simulink model "OscillatorAndLockin_DynamicFreqMod"  (R2022b)
settings: Solver=VariableStepAuto  StartTime=0.0  StopTime=0.1  RelTol=1e-3
model workspace: external: MAT-File C:\Users\yoni\Documents\MATLAB\Examples\AFM\Dynamic Mode\sampledistanceLJ.mat (data not in the file)
undefined symbols (not defined in the file or in its folder): D, I, N, P
libraries: simulink x8, slpidlib x3, simulink_extras x1
Description:
  | A model of the workings of "Non-contant AFM (Atomic Force Microscopy)" aka "Dynamic mode AFM" aka "FrequencyModulated AFM" (FM-AFM)
  | 
  | This model contains:
  | a model of an AFM tip made of a tuning fork with tip-sample interaction force  i.e. a damped harmonic oscillator with external forces applied.
  | a model of an "auto-resonance" circuitry. produces positive and negative force pulses at certain phases of the tip's oscillations.
  | a model of a "Lock-in Amplifier" with PLL mechanism that tracks the oscillator frequency.
  | 
  | The oscillator is driven at it's own resonance frequency with a constant amplitude.
  | This is done by a controlled positive feedback loop, Autoresonance's force is amplified by a value designed to keep amplitude constant.
  | (using a PID and the Lock-in amplitude estimation)
  | 
  | The lock-in and PLL model uses the lock-in calculated phase and use that value to correct the lock-in's internal frequency
  | so it will match the external oscillator's frequency. (using another PID)
settings Model: PacingRate=1000  VariantFading=off  Creator=Yoni Cohen  LastModifiedBy=yoni
settings ConfigSet: Description=Current Conf
settings SolverCC: AlgebraicLoopSolver=LineSearch
settings DebuggingCC: UnconnectedInputMsg=warning  UnconnectedOutputMsg=warning  UnconnectedLineMsg=warning  UniqueDataStoreMsg=error  SFMachineParentedDataDiag=warning
settings HardwareCC: TargetBitPerPointer=64  TargetBitPerSizeT=64  TargetBitPerPtrDiffT=64  TargetLargestAtomicFloat=Float  TargetIntDivRoundTo=Zero  TargetEndianess=LittleEndian  TargetWordSize=64  TargetHWDeviceType=Intel->x86-64 (Windows64)  ProdEqTarget=off
settings ModelReferenceCC: EnableRefExpFcnMdlSchedulingChecks=on
settings SFSimCC: CustomCodeUndefinedFunction=UseInterfaceOnly

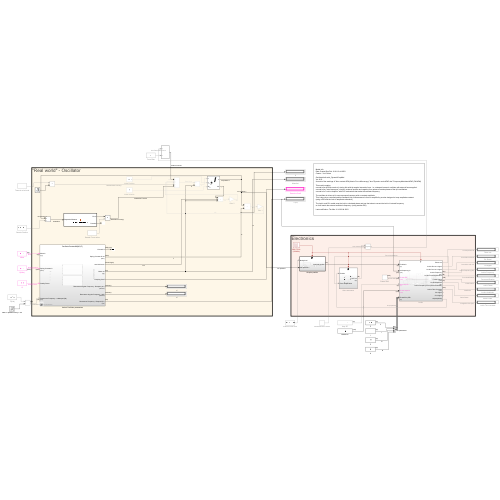
[thumbnail: Simulink's stored preview of the top-level diagram]
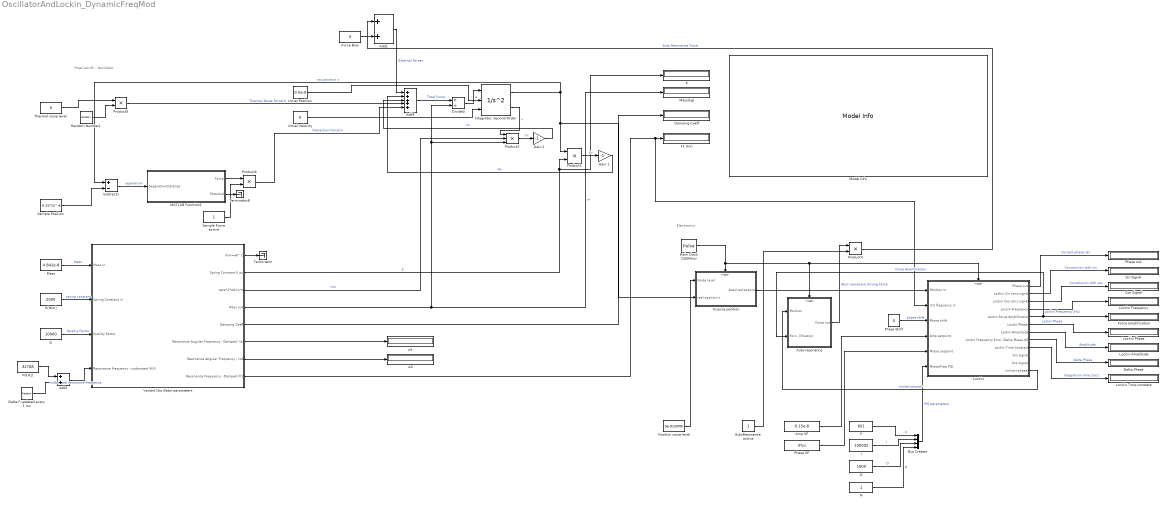
== system OscillatorAndLockin_DynamicFreqMod ==
  note: "Real world" - Oscillator
  note: Electronics
  Acquire position : Subsystem
  Add1 : Sum
  Add2 : Sum
  Add4 : Sum  Inputs=+++++
  Amp SP : Constant  Value=0.15e-8  VectorParams1D=off  SampleTime=-1
  Auto-resonance : Subsystem
  AutoResonance active : Constant  SampleTime=-1
  Bus Creator : BusCreator  Inputs=P,I,D,N
  Cos Signal : Display
  D : Constant  Value=1600  SampleTime=-1
  Damping Coeff : Display
  Delta F updated every 1 ms : RandomNumber  Variance=10  Seed=7546745  SampleTime=1e-3
  Delta Phase : Display
  Divide3 : Product  Inputs=*/
  F0(Hz) : Constant  Value=32768  SampleTime=-1
  F1 (Hz) : Display
  Force Bias : Constant  Value=0  VectorParams1D=off  SampleTime=-1
  Force amplification : Display
  Gain 1 : Gain  Gain=-1
  Gain 2 : Gain  Gain=-1
  I : Constant  Value=100002  SampleTime=-1
  Initial Position : Constant  Value=0.5e-9  VectorParams1D=off
  Initial Velocity : Constant  Value=0
  "Integrator, Second-Order" : SecondOrderIntegrator  ICSourceX=external  LimitX=on  UpperLimitX=0.01  LowerLimitX=-0.01  ICSourceDXDT=external
  K : Display
  K(N/m) : Constant  Value=2000
  Lockin : Subsystem
  Lockin Amplitude : Display
  Lockin Frequency : Display
  Lockin Phase : Display
  Lockin Time constant : Display
  MATLAB Function1 : MATLAB Function  TreatAsAtomicUnit=on
  Main Clock (100MHz) : DiscretePulseGenerator  PulseType=Time based  Period=10^-8  PulseWidth=50
  Mass : Constant  Value=4.842e-8
  Mass(kg) : Display
  Model Info : simulink/Model-Wide Utilities/Model Info  Frame=on  DisplayStringWithTags=|  HorizontalTextAlignment=Left  LeftAlignmentValue=0.02
      | Model Info
      | Date Created %<Created>
      | Creator : %<Creator>
      | %<ModifiedComment>
      | %<ModelName> 
      | Ver. %<ModelVersion>
      | %<Description>
      | Last modification: %<LastModificationDate>
  N : Constant  SampleTime=-1
  P : Constant  Value=601  SampleTime=-1
  Phase SP : Constant  Value=0*pi  SampleTime=-1
  Phase Shift : Constant  Value=0  VectorParams1D=off  SampleTime=-1
  Phase out : Display
  Position noise level : Constant  Value=0e-9/10000  VectorParams1D=off  SampleTime=-1
  Product{1,4..6} (4 alike) : Product
  Product2 : Product  Inputs=3
  Q : Constant  Value=10000
  Random Number1 : RandomNumber  Seed=754666  SampleTime=10^-8
  Sample Force active : Constant  SampleTime=-1
  Sample Position : Constant  Value=-0.25*10^-6  SampleTime=-1
  Sin Signal : Display
  Subtract1 : Sum  Inputs=+-  OutMin=[0]  RndMeth=Nearest
  Terminator : Terminator
  Terminator8 : Terminator
  Thermal noise level : Constant  Value=0  VectorParams1D=off  SampleTime=-1
  Variant Oscillator parameters : Subsystem  Variant=on  VariantControlMode=label  LabelModeActiveChoice=OscillatorTypeVar==1  PropagateVariantConditions=on
  w0 : Display
  w1 : Display
  wires:
  "Integrator, Second-Order"/1 -> Acquire position/2(real position x), Product1/1, Subtract1/1  "osc position x"
  "Integrator, Second-Order"/2 -> Product2/1  "v"
  Product2/1 -> Gain 2/1  "Cv"
  Product1/1 -> Gain 1/1  "Kx"
  Initial Position/1 -> "Integrator, Second-Order"/2
  Initial Velocity/1 -> "Integrator, Second-Order"/3
  Main Clock (100MHz)/1 -> Lockin/Trigger, Auto-resonance/Trigger, Acquire position/Trigger
  Divide3/1 -> "Integrator, Second-Order"/1  "a"
  Auto-resonance/1(Force out) -> Product4/1  "Auto resosnace driving Force"
  Phase Shift/1 -> Lockin/3(Phase shift)  "phase shift"
  Amp SP/1 -> Lockin/4(Amp setpoint)
  F0(Hz)/1 -> Add2/1
  Lockin/5(Lockin Force Amplification) -> Auto-resonance/2(Force Amplification), Force amplification/1  "Force Amplification"
  AutoResonance active/1 -> Product4/2
  Random Number1/1 -> Product5/2
  Thermal noise level/1 -> Product5/1
  Product5/1 -> Add4/4  "Thermal Noise Force(t)"
  Add1/1 -> Add4/1  "External Forces"
  Sample Force active/1 -> Product6/2
  MATLAB Function1/1(Force) -> Product6/1
  Product6/1 -> Add4/5  "Interaction Force(x)"
  Subtract1/1 -> MATLAB Function1/1(SeparationDistance)  "separation"
  K(N/m)/1 -> Variant Oscillator parameters/2(Spring Constant in)  "spring constant"
  Q/1 -> Variant Oscillator parameters/3(Quality Factor)  "Quality Factor"
  Add2/1 -> Variant Oscillator parameters/4(Resonance Frequency - undamped (fr0))  "undamped resonance frequence"
  Variant Oscillator parameters/6(Resonance Angular Frequency - Damped- (w1)) -> w1/1
  Variant Oscillator parameters/8(Resonance Frequency - Damped (fr1)) -> Lockin/2(Init frequency in), F1 (Hz)/1
  Variant Oscillator parameters/4(Mass out) -> Product2/3, Divide3/2, Mass(kg)/1  "m"
  Variant Oscillator parameters/2(Spring Constant K out) -> Product1/2, K/1  "K"
  Variant Oscillator parameters/5(Damping Coeff) -> Damping Coeff/1
  Variant Oscillator parameters/3(zeta*2*w0=c/m) -> Product2/2  "c/m"
  Variant Oscillator parameters/7(Resonance Angular Frequency - (w0)) -> w0/1
  Mass/1 -> Variant Oscillator parameters/1(Mass in)  "Mass"
  Add4/1 -> Divide3/1  "Total Force"
  Gain 1/1 -> Add4/2  "-Kx"
  Gain 2/1 -> Add4/3  "-Cv"
  Variant Oscillator parameters/1(K/m=w0^2) -> Terminator/1
  Lockin/1(Phase out) -> Phase out/1  "Current phase val"
  Lockin/3(Lockin Cos conv signal) -> Cos Signal/1  "Convolution with cos"
  Lockin/4(Lockin Frequency) -> Lockin Frequency/1  "Lockin Frequency [Hz]"
  Lockin/6(Lockin Phase) -> Lockin Phase/1  "Lockin Phase"
  Lockin/8(Lockin Frequency Error (Delta Phase diff)) -> Delta Phase/1  "Delta Phase"
  Lockin/9(Lockin Time Constant) -> Lockin Time constant/1  "Integration time [sec]"
  MATLAB Function1/2(Potential) -> Terminator8/1
  Lockin/7(Lockin Amplitude) -> Lockin Amplitude/1  "Amplitude"
  Lockin/2(Lockin Sin conv signal) -> Sin Signal/1  "Convolution with sin"
  Force Bias/1 -> Add1/2
  Delta F updated every 1 ms/1 -> Add2/2
  Sample Position/1 -> Subtract1/2
  Acquire position/1(Acquired position) -> Lockin/1(Position in)
  Position noise level/1 -> Acquire position/1(Noise level)
  Phase SP/1 -> Lockin/5(Phase setpoint)
  I/1 -> Bus Creator/2  "I"
  D/1 -> Bus Creator/3  "D"
  P/1 -> Bus Creator/1  "P"
  N/1 -> Bus Creator/4  "N"
  Bus Creator/1 -> Lockin/6(Phase/Freq PID)  "PID parameters"
  Lockin/12(sin(wt+phase)) -> Auto-resonance/1(Position)  "sin(wt+phase)"
  Product4/1 -> Add1/1  "Auto Resonance Force"

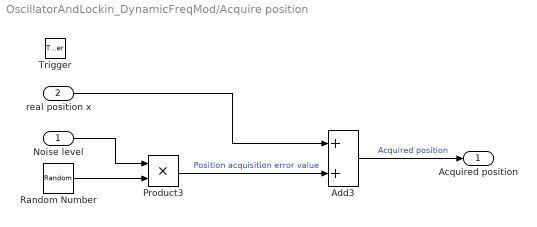
== system OscillatorAndLockin_DynamicFreqMod/Acquire position ==
  Noise level : Inport
  real position x : Inport  Port=2
  Trigger : TriggerPort  VariantControl=Variant  PortDimensions=1
  Add3 : Sum
  Product3 : Product
  Random Number : RandomNumber  Seed=7546767
  Acquired position : Outport  VectorParamsAs1DForOutWhenUnconnected=off
  wires:
  Product3/1 -> Add3/2  "Position acquisition error value"
  Random Number/1 -> Product3/2
  Noise level/1 -> Product3/1
  Add3/1 -> Acquired position/1  "Acquired position"
  real position x/1 -> Add3/1

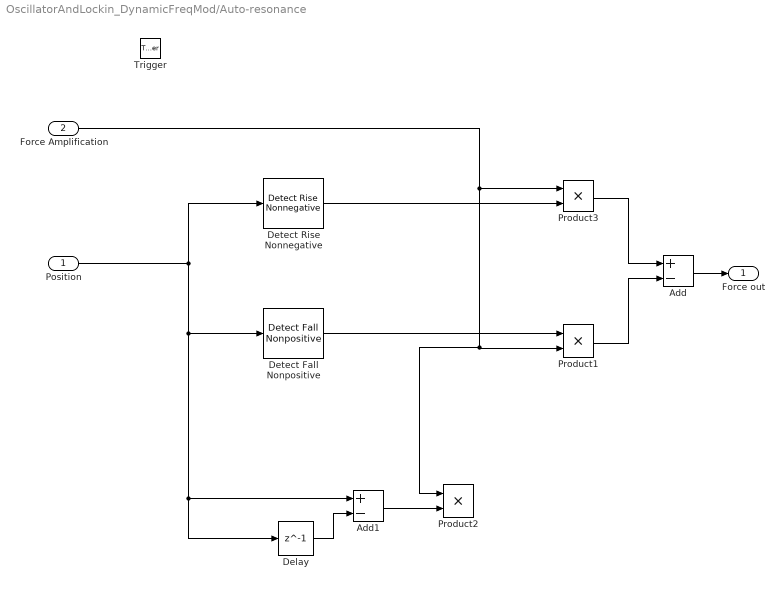
== system OscillatorAndLockin_DynamicFreqMod/Auto-resonance ==
  Position : Inport
  Force Amplification : Inport  Port=2
  Trigger : TriggerPort  VariantControl=Variant  PortDimensions=1
  Add : Sum  Inputs=+-
  Add1 : Sum  Inputs=+-
  Delay : Delay  DelayLength=1  InitialCondition=0
  Detect Fall Nonpositive : simulink/Logic and Bit Operations/Detect Fall Nonpositive  vinit=0  OutDataTypeStr=boolean
  Detect Rise Nonnegative : simulink/Logic and Bit Operations/Detect Rise Nonnegative  vinit=0  OutDataTypeStr=uint8
  Product1 : Product
  Product2 : Product
  Product3 : Product
  Force out : Outport  Unit=N  VectorParamsAs1DForOutWhenUnconnected=off
  wires:
  Position/1 -> Detect Rise Nonnegative/1, Add1/1, Delay/1, Detect Fall Nonpositive/1
  Detect Rise Nonnegative/1 -> Product3/2
  Force Amplification/1 -> Product3/1, Product2/1, Product1/2
  Detect Fall Nonpositive/1 -> Product1/1
  Product1/1 -> Add/2
  Product3/1 -> Add/1
  Delay/1 -> Add1/2
  Add1/1 -> Product2/2
  Add/1 -> Force out/1

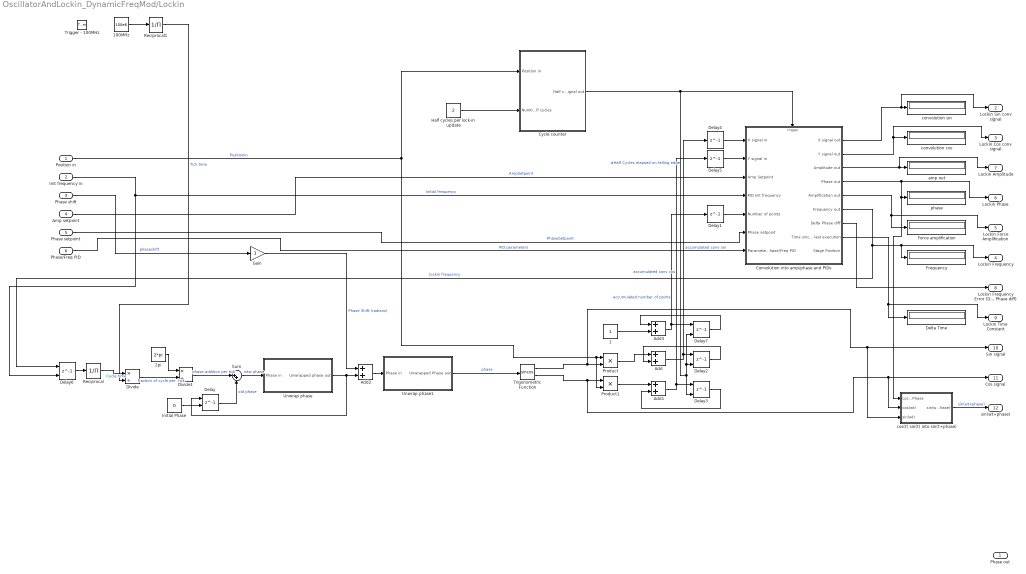
== system OscillatorAndLockin_DynamicFreqMod/Lockin ==
  Position in : Inport  Unit=m
  Init frequency in : Inport  Port=2  Unit=Hz
  Phase shift : Inport  Port=3  OutMin=[-2]  OutMax=[2]  Unit=rad
  Amp setpoint : Inport  Port=4  Unit=m
  Phase setpoint : Inport  Port=5  OutMin=[-2]  OutMax=[2]  Unit=rad
  Phase/Freq PID : Inport  Port=6  Unit=m
  Trigger - 100MHz : TriggerPort  VariantControl=Variant  ShowOutputPort=on  PortDimensions=1
  1 : Constant  OutDataTypeStr=Inherit: Inherit via back propagation
  100MHz : Constant  Value=100e6  OutDataTypeStr=Inherit: Inherit via back propagation
  2pi : Constant  Value=2*pi  OutDataTypeStr=Inherit: Inherit via back propagation
  Add{,1..3} (4 alike) : Sum
  Convolution into amp/phase and PIDs : Subsystem
  Cycle counter : Subsystem
  Delay : Delay  DelayLength=1  InitialConditionSource=Input port  InitialCondition=0
      settings: InputPortMap=u0,p4
  Delay1 : Delay  DelayLength=1  InitialCondition=0
  Delay2 : Delay  DelayLength=1  InitialCondition=0  ExternalReset=Falling
      settings: InputPortMap=u0,r5
  Delay3 : Delay  DelayLength=1  InitialCondition=0  ExternalReset=Falling
      settings: InputPortMap=u0,r5
  Delay4 : Delay  DelayLength=1  InitialCondition=0
  Delay5 : Delay  DelayLength=1  InitialCondition=0
  Delay6 : Delay  DelayLength=1  InitialConditionSource=Input port  InitialCondition=0
      settings: InputPortMap=u0,p4
  Delay7 : Delay  DelayLength=1  InitialCondition=0  ExternalReset=Falling
      settings: InputPortMap=u0,r5
  Delta Time : Display
  Divide : Product  Inputs=*/
  Divide1 : Product  Inputs=*/
  Force amplification : Display
  Frequency : Display
  Gain : Gain
  Half cycles per lock-in update : Constant  Value=2  OutDataTypeStr=Inherit: Inherit via back propagation  SampleTime=-1
  Initial Phase : Constant  Value=0  OutDataTypeStr=Inherit: Inherit via back propagation
  Product : Product
  Product1 : Product
  Reciprocal : Product  Inputs=/
  Reciprocal1 : Product  Inputs=/
  Sum : Sum  Inputs=|++
  Trigonometric Function : Trigonometry  Operator=sincos  ApproximationMethod=CORDIC  NumberOfIterations=64
  Unwrap phase : Subsystem
  Unwrap phase1 : Subsystem
  amp out : Display
  convolution cos : Display
  convolution sin : Display
  cos(t) sin(t) into sin(t+phase) : Subsystem
  phase : Display
  Phase out : Outport  VectorParamsAs1DForOutWhenUnconnected=off
  Lockin Sin conv signal : Outport  Port=2  VectorParamsAs1DForOutWhenUnconnected=off
  Lockin Cos conv signal : Outport  Port=3  VectorParamsAs1DForOutWhenUnconnected=off
  Lockin Frequency : Outport  Port=4  Unit=Hz  InitialOutput=[32769]  VectorParamsAs1DForOutWhenUnconnected=off
  Lockin Force Amplification : Outport  Port=5  VectorParamsAs1DForOutWhenUnconnected=off
  Lockin Phase : Outport  Port=6  Unit=rad  VectorParamsAs1DForOutWhenUnconnected=off
  Lockin Amplitude : Outport  Port=7  Unit=m  VectorParamsAs1DForOutWhenUnconnected=off
  Lockin Frequency Error (Delta Phase diff) : Outport  Port=8  VectorParamsAs1DForOutWhenUnconnected=off
  Lockin Time Constant : Outport  Port=9  Unit=sec  VectorParamsAs1DForOutWhenUnconnected=off
  Sin signal : Outport  Port=10  VectorParamsAs1DForOutWhenUnconnected=off
  Cos signal : Outport  Port=11  VectorParamsAs1DForOutWhenUnconnected=off
  sin(wt+phase) : Outport  Port=12  VectorParamsAs1DForOutWhenUnconnected=off
  wires:
  Divide/1 -> Divide1/2  "fraction of cycle per  tick"
  2pi/1 -> Divide1/1
  Reciprocal/1 -> Divide/1  "Cycle time"
  Trigonometric Function/1 -> Product/2, cos(t) sin(t) into sin(t+phase)/3(sin(wt)), Sin signal/1
  Trigonometric Function/2 -> Product1/1, cos(t) sin(t) into sin(t+phase)/2(cos(wt)), Cos signal/1
  Reciprocal1/1 -> Divide/2  "Tick time"
  Position in/1 -> Cycle counter/1(Position in), Product1/2, Product/1  "Positionin"
  Delay3/1 -> Add1/2
  Delay/1 -> Sum/2  "old phase"
  Delay2/1 -> Add/2
  Convolution into amp/phase and PIDs/3(Amplitude out) -> Lockin Amplitude/1, amp out/1
  Convolution into amp/phase and PIDs/1(X signal out) -> convolution sin/1, Lockin Sin conv signal/1
  Convolution into amp/phase and PIDs/2(Y signal out) -> Lockin Cos conv signal/1, convolution cos/1
  Add/1 -> Delay4/1, Delay2/1  "accumulated conv sin"
  Add1/1 -> Delay3/1, Delay5/1  "accumulated conv cos"
  Divide1/1 -> Sum/1  "phase addition per tick"
  Amp setpoint/1 -> Convolution into amp/phase and PIDs/3(Amp Setpoint)  "AmpSetpoint"
  Convolution into amp/phase and PIDs/5(Amplification out) -> Lockin Force Amplification/1, Force amplification/1
  Init frequency in/1 -> Delay6/2, Convolution into amp/phase and PIDs/4(PID Init frequency)  "Initial frequency"
  Delay6/1 -> Reciprocal/1
  Unwrap phase/1(Unwrapped phase out) -> Delay/1, Add2/2
  Sum/1 -> Unwrap phase/1(Phase in)  "new phase"
  Add2/1 -> Unwrap phase1/1(Phase in)
  Unwrap phase1/1(Unwrapped Phase out) -> Trigonometric Function/1  "phase"
  Half cycles per lock-in update/1 -> Cycle counter/2(Number of half cycles)
  Gain/1 -> Add2/1  "Phase Shift (radians)"
  Convolution into amp/phase and PIDs/4(Phase out) -> Lockin Phase/1, cos(t) sin(t) into sin(t+phase)/1(Lockin Phase), phase/1
  Convolution into amp/phase and PIDs/6(Frequency out) -> Delay6/1, Frequency/1, Lockin Frequency/1  "lockin frequency"
  Convolution into amp/phase and PIDs/7(Delta Phase diff) -> Lockin Frequency Error (Delta Phase diff)/1
  Convolution into amp/phase and PIDs/8(Time since last execution) -> Lockin Time Constant/1, Delta Time/1
  Product1/1 -> Add1/1
  Product/1 -> Add/1
  Delay5/1 -> Convolution into amp/phase and PIDs/2(Y signal in)
  Delay4/1 -> Convolution into amp/phase and PIDs/1(X signal in)
  Cycle counter/1(Half cycle counter signal out) -> Convolution into amp/phase and PIDs/Trigger, Delay7/2, Delay2/2, Delay3/2  "#Half Cycles elapsed on falling edge"
  Add3/1 -> Delay1/1, Delay7/1  "accumulated number of points"
  Delay7/1 -> Add3/1
  1/1 -> Add3/2
  Delay1/1 -> Convolution into amp/phase and PIDs/5(Number of points)
  Phase shift/1 -> Gain/1  "phaseshift"
  Phase setpoint/1 -> Convolution into amp/phase and PIDs/6(Phase setpoint)  "PhaseSetpoint"
  100MHz/1 -> Reciprocal1/1
  Phase/Freq PID/1 -> Convolution into amp/phase and PIDs/7(Parameters Phase/Freq PID)  "PID parameters"
  Initial Phase/1 -> Delay/2
  cos(t) sin(t) into sin(t+phase)/1(sin(wt+phase)) -> sin(wt+phase)/1  "sin(wt+phase)"

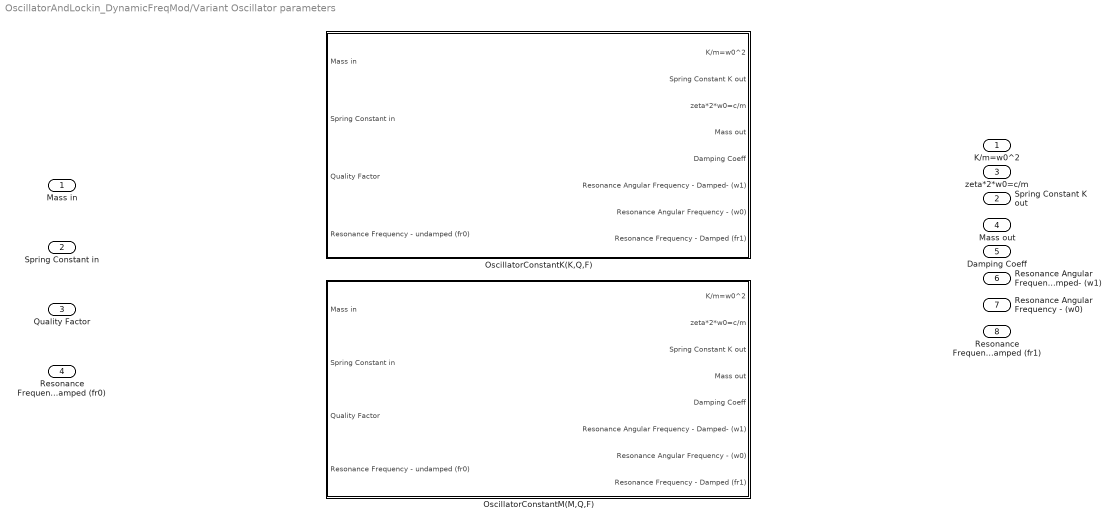
== system OscillatorAndLockin_DynamicFreqMod/Variant Oscillator parameters ==
  Mass in : Inport  Unit=kg
  Spring Constant in : Inport  Port=2  Unit=N/m
  Quality Factor : Inport  Port=3
  Resonance Frequency - undamped (fr0) : Inport  Port=4  Unit=Hz
  OscillatorConstantK(K,Q,F) : Subsystem  VariantControl=OscillatorTypeVar==0
  OscillatorConstantM(M,Q,F) : Subsystem  VariantControl=OscillatorTypeVar==1
  K/m=w0^2 : Outport  VectorParamsAs1DForOutWhenUnconnected=off
  Spring Constant K out : Outport  Port=2  Unit=N/m  VectorParamsAs1DForOutWhenUnconnected=off
  zeta*2*w0=c/m : Outport  Port=3  VectorParamsAs1DForOutWhenUnconnected=off
  Mass out : Outport  Port=4  Unit=kg  VectorParamsAs1DForOutWhenUnconnected=off
  Damping Coeff : Outport  Port=5  VectorParamsAs1DForOutWhenUnconnected=off
  Resonance Angular Frequency - Damped- (w1) : Outport  Port=6  Unit=rad/sec  VectorParamsAs1DForOutWhenUnconnected=off
  Resonance Angular Frequency - (w0) : Outport  Port=7  Unit=rad/sec  VectorParamsAs1DForOutWhenUnconnected=off
  Resonance Frequency - Damped (fr1) : Outport  Port=8  Unit=Hz  VectorParamsAs1DForOutWhenUnconnected=off

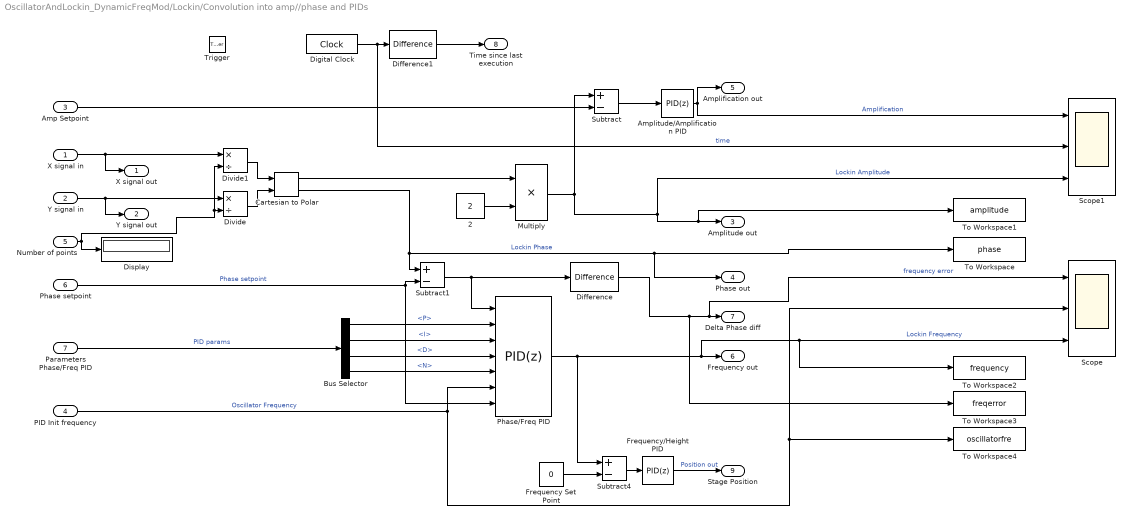
== system OscillatorAndLockin_DynamicFreqMod/Lockin/Convolution into amp//phase and PIDs ==
  X signal in : Inport
  Y signal in : Inport  Port=2
  Amp Setpoint : Inport  Port=3
  PID Init frequency : Inport  Port=4
  Number of points : Inport  Port=5
  Phase setpoint : Inport  Port=6
  Parameters Phase/Freq PID : Inport  Port=7
  Trigger : TriggerPort  TriggerType=falling  VariantControl=Variant  PortDimensions=1
  2 : Constant  Value=2  VectorParams1D=off  SampleTime=-1
  Amplitude/Amplification PID : slpidlib/PID Controller  Controller=PID  Form=Parallel  TimeDomain=Discrete-time  UseExternalTs=off  SampleTime=-1  IntegratorMethod=Trapezoidal  FilterMethod=Trapezoidal  ControllerParametersSource=internal  P=-45000  I=-350000000  UseKiTs=off  D=-10000  N=10  UseFilter=on  TunerSelectOption=Frequency Response Based  InitialConditionSource=internal  InitialConditionForIntegrator=0  InitialConditionForFilter=0  DifferentiatorICPrevScaledInput=0  ExternalReset=none  TrackingMode=off  Kt=1  LimitOutput=off  SatLimitsSource=internal  UpperSaturationLimit=inf  LowerSaturationLimit=-inf  LinearizeAsGain=off  AntiWindupMode=none  Kb=1  LimitIntegrator=off  UpperIntegratorSaturationLimit=inf  LowerIntegratorSaturationLimit=-inf  RndMeth=Round  POutMin=[]  POutMax=[]  IOutMin=[]  IOutMax=[]  DOutMin=[]  DOutMax=[]  NOutMin=[]  NOutMax=[]  SumOutMin=[]  SumOutMax=[]  SaturationOutMin=[]  SaturationOutMax=[]  PParamMin=[]  PParamMax=[]  IParamMin=[]  IParamMax=[]  DParamMin=[]  DParamMax=[]  NParamMin=[]  NParamMax=[]  KbParamMin=[]  KbParamMax=[]  KtParamMin=[]  KtParamMax=[]  KbOutMin=[]  KbOutMax=[]  KtOutMin=[]  KtOutMax=[]  IntegratorOutMin=[]  IntegratorOutMax=[]  FilterOutMin=[]  FilterOutMax=[]  SumI1OutMin=[]  SumI1OutMax=[]  SumI2OutMin=[]  SumI2OutMax=[]  SumI3OutMin=[]  SumI3OutMax=[]  SumI4OutMin=[]  SumI4OutMax=[]  SumDOutMin=[]  SumDOutMax=[]  DifferentiatorOutMin=[]  DifferentiatorOutMax=[]  FilterDiffOutCoefMin=[]  FilterDiffOutCoefMax=[]  ReciprocalOutMin=[]  ReciprocalOutMax=[]  SumDenOutMin=[]  SumDenOutMax=[]  SumNumOutMin=[]  SumNumOutMax=[]  DivideOutMin=[]  DivideOutMax=[]  UdiffTsProdOutMin=[]  UdiffTsProdOutMax=[]  NTsProdOutMin=[]  NTsProdOutMax=[]  UintegralTsProdOutMin=[]  UintegralTsProdOutMax=[]  UngainTsProdOutMin=[]  UngainTsProdOutMax=[]  ClampingZeroOutDataTypeStr=Inherit: Inherit via back propagation  ClampingZeroOutMin=[]  ClampingZeroOutMax=[]  FilterDenConstantOutDataTypeStr=Inherit: Inherit via back propagation  FilterDenConstantOutMin=[]  FilterDenConstantOutMax=[]  PCopyOutDataTypeStr=Inherit: Inherit via back propagation  PCopyOutMin=[]  PCopyOutMax=[]  NCopyOutDataTypeStr=Inherit: Inherit via back propagation  NCopyOutMin=[]  NCopyOutMax=[]  IntegratorContinuousStateAttributes=''  IntegratorStateMustResolveToSignalObject=off  IntegratorRTWStateStorageClass=Auto  FilterContinuousStateAttributes=''  FilterStateMustResolveToSignalObject=off  FilterRTWStateStorageClass=Auto  ParallelPVariant=InternalParameters  IdealPVariant=Disabled  IVariant=InternalParameters  DVariant=InternalParameters  IntegratorVariant=Discrete  SatVariant=Disabled  AWVariant=Passthrough  PCopyVariant=Disabled  TRVariant=Disabled  FdbkBlocksVariant=Forward  IdealPFdbkVariant=Disabled  SatFdbkVariant=Disabled  DerivativeFilterVariant=TrapezoidalFilter  NVariant=InternalParameters  NCopyVariant=InternalParameters  FilterICVariant=InternalICsFilter  IntegratorICVariant=InternalICs  ExternalResetVariant=Disabled  TRSumVariant=Passthrough  SumFdbkVariant=Disabled  SumVariant=Sum_PID  TsampFilterVariant=InternalTs  TsampNgainVariant=Passthrough  TsampIntegralVariant=Passthrough  ExternalSaturationOutDataTypeStr=Inherit: Same as second input
  Bus Selector : BusSelector  OutputSignals=P,I,D,N
  Cartesian to Polar : simulink_extras/Transformations/Cartesian to Polar
  Difference : simulink/Quick Insert/Discrete/Difference  ICPrevInput=0.0  OutMin=[]  OutMax=[]  OutDataType=fixdt(1, 16)  OutScaling=2^-10  DoSatur=off
  Difference1 : simulink/Quick Insert/Discrete/Difference  ICPrevInput=0.0  OutMin=[]  OutMax=[]  OutDataType=fixdt(1, 16)  OutScaling=2^-10  DoSatur=off
  Digital Clock : DigitalClock  SampleTime=-1
  Display : Display
  Divide : Product  Inputs=*/
  Divide1 : Product  Inputs=*/
  Frequency Set Point : Constant  Value=0  SampleTime=-1
  Frequency/Height PID : slpidlib/PID Controller  Controller=PID  Form=Parallel  TimeDomain=Discrete-time  UseExternalTs=off  SampleTime=-1  IntegratorMethod=Forward Euler  FilterMethod=Forward Euler  ControllerParametersSource=internal  P=1  I=1  UseKiTs=off  D=0  N=100  UseFilter=on  TunerSelectOption=Transfer Function Based (PID Tuner App)  InitialConditionSource=internal  InitialConditionForIntegrator=0  InitialConditionForFilter=0  DifferentiatorICPrevScaledInput=0  ExternalReset=none  TrackingMode=off  Kt=1  LimitOutput=off  SatLimitsSource=internal  UpperSaturationLimit=inf  LowerSaturationLimit=-inf  LinearizeAsGain=off  AntiWindupMode=none  Kb=1  LimitIntegrator=off  UpperIntegratorSaturationLimit=inf  LowerIntegratorSaturationLimit=-inf  POutMin=[]  POutMax=[]  IOutMin=[]  IOutMax=[]  DOutMin=[]  DOutMax=[]  NOutMin=[]  NOutMax=[]  SumOutMin=[]  SumOutMax=[]  SaturationOutMin=[]  SaturationOutMax=[]  PParamMin=[]  PParamMax=[]  IParamMin=[]  IParamMax=[]  DParamMin=[]  DParamMax=[]  NParamMin=[]  NParamMax=[]  KbParamMin=[]  KbParamMax=[]  KtParamMin=[]  KtParamMax=[]  KbOutMin=[]  KbOutMax=[]  KtOutMin=[]  KtOutMax=[]  IntegratorOutMin=[]  IntegratorOutMax=[]  FilterOutMin=[]  FilterOutMax=[]  SumI1OutMin=[]  SumI1OutMax=[]  SumI2OutMin=[]  SumI2OutMax=[]  SumI3OutMin=[]  SumI3OutMax=[]  SumI4OutMin=[]  SumI4OutMax=[]  SumDOutMin=[]  SumDOutMax=[]  DifferentiatorOutMin=[]  DifferentiatorOutMax=[]  FilterDiffOutCoefMin=[]  FilterDiffOutCoefMax=[]  ReciprocalOutMin=[]  ReciprocalOutMax=[]  SumDenOutMin=[]  SumDenOutMax=[]  SumNumOutMin=[]  SumNumOutMax=[]  DivideOutMin=[]  DivideOutMax=[]  UdiffTsProdOutMin=[]  UdiffTsProdOutMax=[]  NTsProdOutMin=[]  NTsProdOutMax=[]  UintegralTsProdOutMin=[]  UintegralTsProdOutMax=[]  UngainTsProdOutMin=[]  UngainTsProdOutMax=[]  ClampingZeroOutDataTypeStr=Inherit: Inherit via back propagation  ClampingZeroOutMin=[]  ClampingZeroOutMax=[]  FilterDenConstantOutDataTypeStr=Inherit: Inherit via back propagation  FilterDenConstantOutMin=[]  FilterDenConstantOutMax=[]  PCopyOutDataTypeStr=Inherit: Inherit via back propagation  PCopyOutMin=[]  PCopyOutMax=[]  NCopyOutDataTypeStr=Inherit: Inherit via back propagation  NCopyOutMin=[]  NCopyOutMax=[]  IntegratorContinuousStateAttributes=''  IntegratorStateMustResolveToSignalObject=off  IntegratorRTWStateStorageClass=Auto  FilterContinuousStateAttributes=''  FilterStateMustResolveToSignalObject=off  FilterRTWStateStorageClass=Auto  ParallelPVariant=InternalParameters  IdealPVariant=Disabled  IVariant=InternalParameters  DVariant=InternalParameters  IntegratorVariant=Discrete  SatVariant=Disabled  AWVariant=Passthrough  PCopyVariant=Disabled  TRVariant=Disabled  FdbkBlocksVariant=Forward  IdealPFdbkVariant=Disabled  SatFdbkVariant=Disabled  DerivativeFilterVariant=ForwardEulerFilter  NVariant=InternalParameters  NCopyVariant=Disabled  FilterICVariant=InternalICsFilter  IntegratorICVariant=InternalICs  ExternalResetVariant=Disabled  TRSumVariant=Passthrough  SumFdbkVariant=Disabled  SumVariant=Sum_PID  TsampFilterVariant=InternalTs  TsampNgainVariant=Passthrough  TsampIntegralVariant=Passthrough  ExternalSaturationOutDataTypeStr=Inherit: Same as second input
  Multiply : Product  Inputs=**
  Phase/Freq PID : slpidlib/PID Controller  Controller=PID  Form=Parallel  TimeDomain=Discrete-time  UseExternalTs=off  SampleTime=-1  IntegratorMethod=Forward Euler  FilterMethod=Forward Euler  ControllerParametersSource=external  P=20  I=100  UseKiTs=off  D=1400  N=1  UseFilter=on  TunerSelectOption=Transfer Function Based (PID Tuner App)  InitialConditionSource=external  InitialConditionForIntegrator=0  InitialConditionForFilter=0  DifferentiatorICPrevScaledInput=0  ExternalReset=none  TrackingMode=off  Kt=1  LimitOutput=off  SatLimitsSource=internal  UpperSaturationLimit=inf  LowerSaturationLimit=-inf  LinearizeAsGain=off  AntiWindupMode=none  Kb=1  LimitIntegrator=off  UpperIntegratorSaturationLimit=inf  LowerIntegratorSaturationLimit=-inf  POutMin=[]  POutMax=[]  IOutMin=[]  IOutMax=[]  DOutMin=[]  DOutMax=[]  NOutMin=[]  NOutMax=[]  SumOutMin=[]  SumOutMax=[]  SaturationOutMin=[]  SaturationOutMax=[]  PParamMin=[]  PParamMax=[]  IParamMin=[]  IParamMax=[]  DParamMin=[]  DParamMax=[]  NParamMin=[]  NParamMax=[]  KbParamMin=[]  KbParamMax=[]  KtParamMin=[]  KtParamMax=[]  KbOutMin=[]  KbOutMax=[]  KtOutMin=[]  KtOutMax=[]  IntegratorOutMin=[]  IntegratorOutMax=[]  FilterOutMin=[]  FilterOutMax=[]  SumI1OutMin=[]  SumI1OutMax=[]  SumI2OutMin=[]  SumI2OutMax=[]  SumI3OutMin=[]  SumI3OutMax=[]  SumI4OutMin=[]  SumI4OutMax=[]  SumDOutMin=[]  SumDOutMax=[]  DifferentiatorOutMin=[]  DifferentiatorOutMax=[]  FilterDiffOutCoefMin=[]  FilterDiffOutCoefMax=[]  ReciprocalOutMin=[]  ReciprocalOutMax=[]  SumDenOutMin=[]  SumDenOutMax=[]  SumNumOutMin=[]  SumNumOutMax=[]  DivideOutMin=[]  DivideOutMax=[]  UdiffTsProdOutMin=[]  UdiffTsProdOutMax=[]  NTsProdOutMin=[]  NTsProdOutMax=[]  UintegralTsProdOutMin=[]  UintegralTsProdOutMax=[]  UngainTsProdOutMin=[]  UngainTsProdOutMax=[]  ClampingZeroOutDataTypeStr=Inherit: Inherit via back propagation  ClampingZeroOutMin=[]  ClampingZeroOutMax=[]  FilterDenConstantOutDataTypeStr=Inherit: Inherit via back propagation  FilterDenConstantOutMin=[]  FilterDenConstantOutMax=[]  PCopyOutDataTypeStr=Inherit: Inherit via back propagation  PCopyOutMin=[]  PCopyOutMax=[]  NCopyOutDataTypeStr=Inherit: Inherit via back propagation  NCopyOutMin=[]  NCopyOutMax=[]  IntegratorContinuousStateAttributes=''  IntegratorStateMustResolveToSignalObject=off  IntegratorRTWStateStorageClass=Auto  FilterContinuousStateAttributes=''  FilterStateMustResolveToSignalObject=off  FilterRTWStateStorageClass=Auto  ParallelPVariant=ExternalParameters  IdealPVariant=Disabled  IVariant=ExternalParameters  DVariant=ExternalParameters  IntegratorVariant=Discrete  SatVariant=Disabled  AWVariant=Passthrough  PCopyVariant=Disabled  TRVariant=Disabled  FdbkBlocksVariant=Forward  IdealPFdbkVariant=Disabled  SatFdbkVariant=Disabled  DerivativeFilterVariant=ForwardEulerFilter  NVariant=ExternalParameters  NCopyVariant=Disabled  FilterICVariant=ExternalICs  IntegratorICVariant=ExternalICs  ExternalResetVariant=Disabled  TRSumVariant=Passthrough  SumFdbkVariant=Disabled  SumVariant=Sum_PID  TsampFilterVariant=InternalTs  TsampNgainVariant=Passthrough  TsampIntegralVariant=Passthrough  ExternalSaturationOutDataTypeStr=Inherit: Same as second input
  Scope : Scope  NumInputPorts=3
  Scope1 : Scope  NumInputPorts=3
  Subtract : Sum  Inputs=+-
  Subtract1 : Sum  Inputs=+-
  Subtract4 : Sum  Inputs=+-
  To Workspace : ToWorkspace  VariableName=phase  SaveFormat=Timeseries  SampleTime=-1
  To Workspace1 : ToWorkspace  VariableName=amplitude  SaveFormat=Timeseries  SampleTime=-1
  To Workspace2 : ToWorkspace  VariableName=frequency  SaveFormat=Timeseries  SampleTime=-1
  To Workspace3 : ToWorkspace  VariableName=freqerror  SaveFormat=Timeseries  SampleTime=-1
  To Workspace4 : ToWorkspace  VariableName=oscillatorfre  SaveFormat=Timeseries  SampleTime=-1
  X signal out : Outport  VectorParamsAs1DForOutWhenUnconnected=off
  Y signal out : Outport  Port=2  VectorParamsAs1DForOutWhenUnconnected=off
  Amplitude out : Outport  Port=3  Unit=m  VectorParamsAs1DForOutWhenUnconnected=off
  Phase out : Outport  Port=4  Unit=rad  VectorParamsAs1DForOutWhenUnconnected=off
  Amplification out : Outport  Port=5  Unit=N  VectorParamsAs1DForOutWhenUnconnected=off
  Frequency out : Outport  Port=6  Unit=Hz  InitialOutput=[32766]  VectorParamsAs1DForOutWhenUnconnected=off
  Delta Phase diff : Outport  Port=7  Unit=rad  VectorParamsAs1DForOutWhenUnconnected=off
  Time since last execution : Outport  Port=8  Unit=sec  VectorParamsAs1DForOutWhenUnconnected=off
  Stage Position : Outport  Port=9  Unit=m  VectorParamsAs1DForOutWhenUnconnected=off
  wires:
  X signal in/1 -> Divide1/1, X signal out/1
  Y signal in/1 -> Divide/1, Y signal out/1
  Amp Setpoint/1 -> Subtract/2
  Phase/Freq PID/1 -> Frequency out/1, To Workspace2/1, Scope/3, Subtract4/1  "Lockin Frequency"
  PID Init frequency/1 -> To Workspace4/1, Scope/2, Phase/Freq PID/6  "Oscillator Frequency"
  Subtract1/1 -> Phase/Freq PID/1, Difference/1
  Cartesian to Polar/2 -> Subtract1/1, To Workspace/1, Phase out/1  "Lockin Phase"
  Digital Clock/1 -> Scope1/2, Difference1/1  "time"
  Difference1/1 -> Time since last execution/1
  Cartesian to Polar/1 -> Multiply/1
  Multiply/1 -> Scope1/3, To Workspace1/1, Amplitude out/1, Subtract/1  "Lockin Amplitude"
  Subtract/1 -> Amplitude/Amplification PID/1
  Amplitude/Amplification PID/1 -> Amplification out/1, Scope1/1  "Amplification"
  Number of points/1 -> Divide1/2, Divide/2, Display/1
  Divide1/1 -> Cartesian to Polar/1
  2/1 -> Multiply/2
  Phase setpoint/1 -> Subtract1/2, Phase/Freq PID/7  "Phase setpoint"
  Difference/1 -> To Workspace3/1, Scope/1, Delta Phase diff/1  "frequency error"
  Bus Selector/1 -> Phase/Freq PID/2  "<P>"
  Bus Selector/2 -> Phase/Freq PID/3  "<I>"
  Bus Selector/3 -> Phase/Freq PID/4  "<D>"
  Bus Selector/4 -> Phase/Freq PID/5  "<N>"
  Parameters Phase/Freq PID/1 -> Bus Selector/1  "PID params"
  Divide/1 -> Cartesian to Polar/2
  Frequency/Height PID/1 -> Stage Position/1  "Position out"
  Subtract4/1 -> Frequency/Height PID/1
  Frequency Set Point/1 -> Subtract4/2

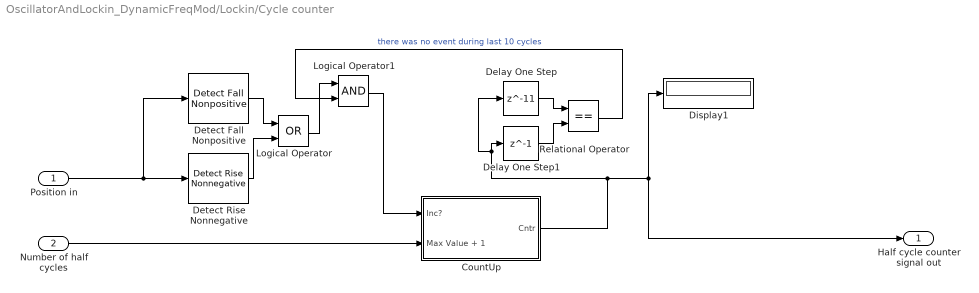
== system OscillatorAndLockin_DynamicFreqMod/Lockin/Cycle counter ==
  Position in : Inport
  Number of half cycles : Inport  Port=2  OutDataTypeStr=uint16
  CountUp : Subsystem
  Delay One Step : Delay  DelayLength=11
  Delay One Step1 : Delay  DelayLength=1
  Detect Fall Nonpositive : simulink/Logic and Bit Operations/Detect Fall Nonpositive  vinit=0  OutDataTypeStr=boolean
  Detect Rise Nonnegative : simulink/Logic and Bit Operations/Detect Rise Nonnegative  vinit=0  OutDataTypeStr=boolean
  Display1 : Display
  Logical Operator : Logic  Operator=OR  AllPortsSameDT=off  OutDataTypeStr=boolean
  Logical Operator1 : Logic  AllPortsSameDT=off  OutDataTypeStr=boolean
  Relational Operator : RelationalOperator  Operator===  OutDataTypeStr=boolean  RndMeth=Simplest  InputSameDT=off
  Half cycle counter signal out : Outport  VectorParamsAs1DForOutWhenUnconnected=off
  wires:
  Detect Rise Nonnegative/1 -> Logical Operator/2
  Number of half cycles/1 -> CountUp/2(Max Value + 1)
  Position in/1 -> Detect Fall Nonpositive/1, Detect Rise Nonnegative/1
  Detect Fall Nonpositive/1 -> Logical Operator/1
  Logical Operator/1 -> Logical Operator1/1
  CountUp/1(Cntr) -> Delay One Step1/1, Delay One Step/1, Display1/1, Half cycle counter signal out/1
  Delay One Step/1 -> Relational Operator/1
  Delay One Step1/1 -> Relational Operator/2
  Relational Operator/1 -> Logical Operator1/2  "there was no event during last 10 cycles"
  Logical Operator1/1 -> CountUp/1(Inc?)

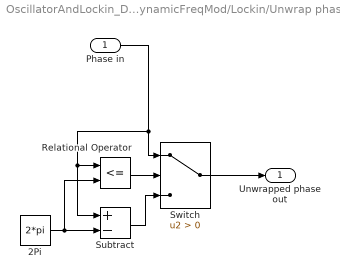
== system OscillatorAndLockin_DynamicFreqMod/Lockin/Unwrap phase ==
  Phase in : Inport  Unit=rad
  2Pi : Constant  Value=2*pi  OutDataTypeStr=Inherit: Inherit via back propagation
  Relational Operator : RelationalOperator  Operator=<=  OutDataTypeStr=boolean  RndMeth=Simplest  InputSameDT=off
  Subtract : Sum  Inputs=+-
  Switch : Switch  Criteria=u2 > Threshold  SaturateOnIntegerOverflow=off  InputSameDT=off
  Unwrapped phase out : Outport  Unit=rad  VectorParamsAs1DForOutWhenUnconnected=off
  wires:
  Relational Operator/1 -> Switch/2
  Phase in/1 -> Switch/1, Relational Operator/1, Subtract/1
  Switch/1 -> Unwrapped phase out/1
  2Pi/1 -> Relational Operator/2, Subtract/2
  Subtract/1 -> Switch/3

== system OscillatorAndLockin_DynamicFreqMod/Lockin/Unwrap phase1 ==
  Phase in : Inport
  Pi : Constant  Value=2*pi  OutDataTypeStr=Inherit: Inherit via back propagation
  Relational Operator : RelationalOperator  Operator=<=  OutDataTypeStr=boolean  RndMeth=Simplest  InputSameDT=off
  Subtract : Sum  Inputs=+-
  Switch : Switch  Criteria=u2 > Threshold  SaturateOnIntegerOverflow=off  InputSameDT=off
  Unwrapped Phase out : Outport  Unit=rad  VectorParamsAs1DForOutWhenUnconnected=off
  wires:
  Relational Operator/1 -> Switch/2
  Phase in/1 -> Switch/1, Relational Operator/1, Subtract/1
  Switch/1 -> Unwrapped Phase out/1
  Pi/1 -> Relational Operator/2, Subtract/2
  Subtract/1 -> Switch/3

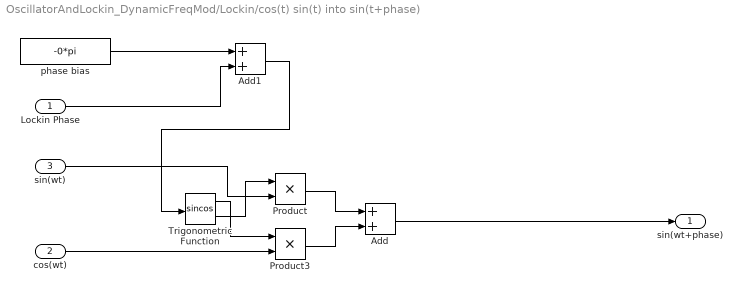
== system OscillatorAndLockin_DynamicFreqMod/Lockin/cos(t) sin(t) into sin(t+phase) ==
  Lockin Phase : Inport  Unit=rad
  cos(wt) : Inport  Port=2
  sin(wt) : Inport  Port=3
  Add : Sum
  Add1 : Sum
  Product : Product
  Product3 : Product
  Trigonometric Function : Trigonometry  Operator=sincos  ApproximationMethod=CORDIC  NumberOfIterations=64
  phase bias : Constant  Value=-0*pi  SampleTime=-1
  sin(wt+phase) : Outport
  wires:
  Trigonometric Function/2 -> Product/1
  Trigonometric Function/1 -> Product3/1
  Product/1 -> Add/1
  sin(wt)/1 -> Product/2
  Product3/1 -> Add/2
  cos(wt)/1 -> Product3/2
  Add/1 -> sin(wt+phase)/1
  phase bias/1 -> Add1/1
  Lockin Phase/1 -> Add1/2
  Add1/1 -> Trigonometric Function/1

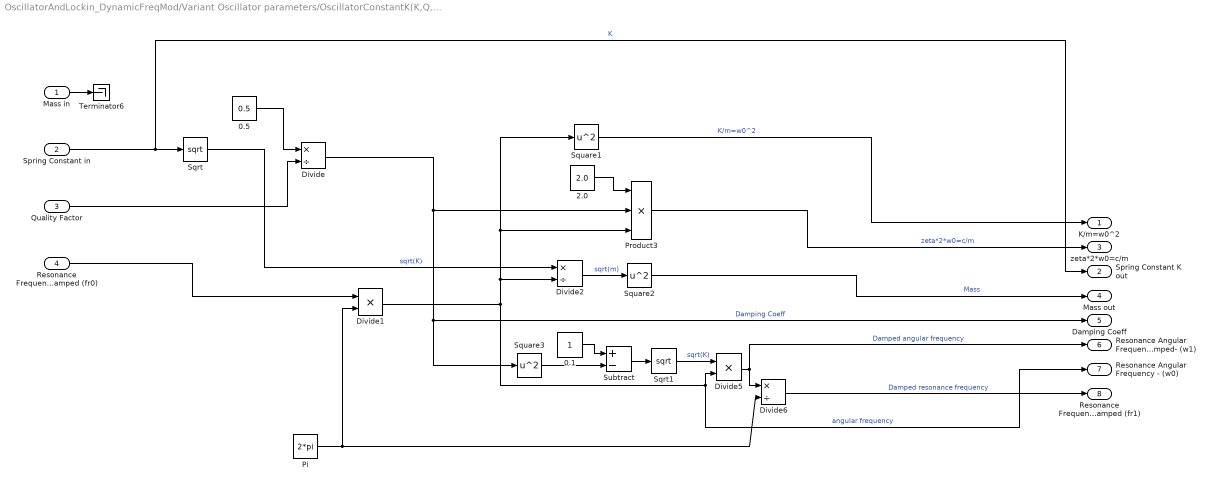
== system OscillatorAndLockin_DynamicFreqMod/Variant Oscillator parameters/OscillatorConstantK(K,Q,F) ==
  Mass in : Inport  Unit=kg
  Spring Constant in : Inport  Port=2  Unit=N/m
  Quality Factor : Inport  Port=3
  Resonance Frequency - undamped (fr0) : Inport  Port=4  Unit=Hz
  0.1 : Constant
  0.5 : Constant  Value=0.5
  2.0 : Constant  Value=2.0
  Divide : Product  Inputs=*/
  Divide1 : Product  Inputs=**
  Divide2 : Product  Inputs=*/
  Divide5 : Product  Inputs=**
  Divide6 : Product  Inputs=*/
  Pi : Constant  Value=2*pi  OutDataTypeStr=Inherit: Inherit via back propagation
  Product3 : Product  Inputs=3
  Sqrt : Sqrt
  Sqrt1 : Sqrt
  Square1 : Math  Operator=square  SignedPower=on
  Square2 : Math  Operator=square  SignedPower=on
  Square3 : Math  Operator=square  SignedPower=on
  Subtract : Sum  Inputs=+-
  Terminator6 : Terminator
  K/m=w0^2 : Outport  VectorParamsAs1DForOutWhenUnconnected=off
  Spring Constant K out : Outport  Port=2  Unit=N/m  VectorParamsAs1DForOutWhenUnconnected=off
  zeta*2*w0=c/m : Outport  Port=3  VectorParamsAs1DForOutWhenUnconnected=off
  Mass out : Outport  Port=4  Unit=kg  VectorParamsAs1DForOutWhenUnconnected=off
  Damping Coeff : Outport  Port=5  VectorParamsAs1DForOutWhenUnconnected=off
  Resonance Angular Frequency - Damped- (w1) : Outport  Port=6  Unit=rad/sec  VectorParamsAs1DForOutWhenUnconnected=off
  Resonance Angular Frequency - (w0) : Outport  Port=7  Unit=rad/sec  VectorParamsAs1DForOutWhenUnconnected=off
  Resonance Frequency - Damped (fr1) : Outport  Port=8  Unit=Hz  VectorParamsAs1DForOutWhenUnconnected=off
  wires:
  Divide1/1 -> Square1/1, Product3/3, Divide2/2, Divide5/2, Resonance Angular Frequency - (w0)/1  "angular frequency"
  Divide5/1 -> Divide6/1, Resonance Angular Frequency - Damped- (w1)/1  "Damped angular frequency"
  0.5/1 -> Divide/1
  Divide2/1 -> Square2/1  "sqrt(m)"
  0.1/1 -> Subtract/1
  Divide/1 -> Square3/1, Damping Coeff/1, Product3/2  "Damping Coeff"
  Square3/1 -> Subtract/2
  Sqrt1/1 -> Divide5/1  "sqrt(K)"
  Subtract/1 -> Sqrt1/1
  Sqrt/1 -> Divide2/1  "sqrt(K)"
  Square1/1 -> K/m=w0^2/1  "K/m=w0^2"
  Pi/1 -> Divide1/2, Divide6/2
  2.0/1 -> Product3/1
  Resonance Frequency - undamped (fr0)/1 -> Divide1/1
  Quality Factor/1 -> Divide/2
  Product3/1 -> zeta*2*w0=c/m/1  "zeta*2*w0=c/m"
  Divide6/1 -> Resonance Frequency - Damped (fr1)/1  "Damped resonance frequency"
  Square2/1 -> Mass out/1  "Mass"
  Spring Constant in/1 -> Spring Constant K out/1, Sqrt/1  "K"
  Mass in/1 -> Terminator6/1

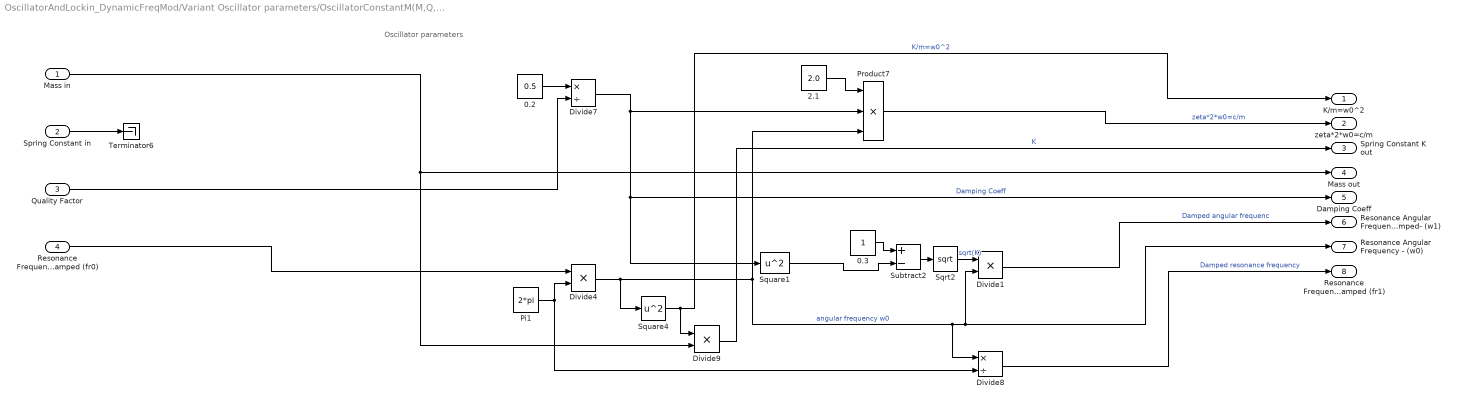
== system OscillatorAndLockin_DynamicFreqMod/Variant Oscillator parameters/OscillatorConstantM(M,Q,F) ==
  note: Oscillator parameters
  Mass in : Inport  Unit=kg
  Spring Constant in : Inport  Port=2  Unit=N/m
  Quality Factor : Inport  Port=3
  Resonance Frequency - undamped (fr0) : Inport  Port=4  Unit=Hz
  0.2 : Constant  Value=0.5
  0.3 : Constant
  2.1 : Constant  Value=2.0
  Divide1 : Product  Inputs=**
  Divide4 : Product  Inputs=**
  Divide7 : Product  Inputs=*/
  Divide8 : Product  Inputs=*/
  Divide9 : Product  Inputs=**
  Pi1 : Constant  Value=2*pi  OutDataTypeStr=Inherit: Inherit via back propagation
  Product7 : Product  Inputs=3
  Sqrt2 : Sqrt
  Square1 : Math  Operator=square  SignedPower=on
  Square4 : Math  Operator=square  SignedPower=on
  Subtract2 : Sum  Inputs=+-
  Terminator6 : Terminator
  K/m=w0^2 : Outport  Unit=N/(kg*m)  VectorParamsAs1DForOutWhenUnconnected=off
  zeta*2*w0=c/m : Outport  Port=2  Unit=N*sec/kg/m  VectorParamsAs1DForOutWhenUnconnected=off
  Spring Constant K out : Outport  Port=3  Unit=N/m  VectorParamsAs1DForOutWhenUnconnected=off
  Mass out : Outport  Port=4  Unit=kg  VectorParamsAs1DForOutWhenUnconnected=off
  Damping Coeff : Outport  Port=5  VectorParamsAs1DForOutWhenUnconnected=off
  Resonance Angular Frequency - Damped- (w1) : Outport  Port=6  Unit=rad/sec  VectorParamsAs1DForOutWhenUnconnected=off
  Resonance Angular Frequency - (w0) : Outport  Port=7  Unit=rad/sec  VectorParamsAs1DForOutWhenUnconnected=off
  Resonance Frequency - Damped (fr1) : Outport  Port=8  Unit=Hz  VectorParamsAs1DForOutWhenUnconnected=off
  wires:
  Resonance Frequency - undamped (fr0)/1 -> Divide4/1
  Sqrt2/1 -> Divide1/1  "sqrt(K)"
  Square4/1 -> K/m=w0^2/1, Divide9/1  "K/m=w0^2"
  Pi1/1 -> Divide8/2, Divide4/2
  Divide7/1 -> Product7/2, Square1/1, Damping Coeff/1  "Damping Coeff"
  Divide4/1 -> Square4/1, Product7/3, Divide8/1, Resonance Angular Frequency - (w0)/1, Divide1/2  "angular frequency w0"
  Divide1/1 -> Resonance Angular Frequency - Damped- (w1)/1  "Damped angular frequenc"
  2.1/1 -> Product7/1
  Divide8/1 -> Resonance Frequency - Damped (fr1)/1  "Damped resonance frequency"
  Subtract2/1 -> Sqrt2/1
  Square1/1 -> Subtract2/2
  0.2/1 -> Divide7/1
  0.3/1 -> Subtract2/1
  Mass in/1 -> Divide9/2, Mass out/1
  Divide9/1 -> Spring Constant K out/1  "K"
  Product7/1 -> zeta*2*w0=c/m/1  "zeta*2*w0=c/m"
  Quality Factor/1 -> Divide7/2
  Spring Constant in/1 -> Terminator6/1

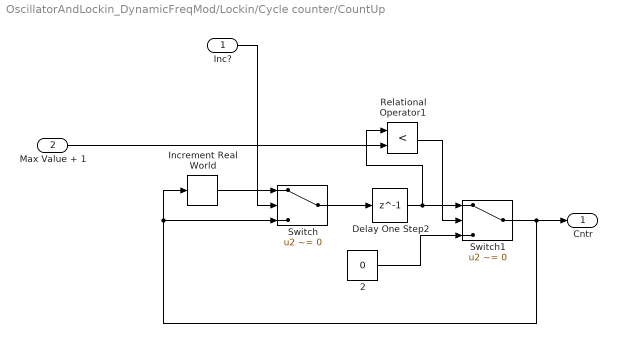
== system OscillatorAndLockin_DynamicFreqMod/Lockin/Cycle counter/CountUp ==
  Inc? : Inport
  Max Value + 1 : Inport  Port=2
  2 : Constant  Value=0  OutDataTypeStr=uint16
  Delay One Step2 : Delay  DelayLength=1
  Increment Real World : simulink/Additional Math & Discrete/Additional Math: Increment - Decrement/Increment Real World
  Relational Operator1 : RelationalOperator  Operator=<  OutDataTypeStr=boolean  RndMeth=Simplest  InputSameDT=off
  Switch : Switch  Criteria=u2 ~= 0  SaturateOnIntegerOverflow=off  InputSameDT=off
  Switch1 : Switch  Criteria=u2 ~= 0  SaturateOnIntegerOverflow=off  InputSameDT=off
  Cntr : Outport  VectorParamsAs1DForOutWhenUnconnected=off
  wires:
  Switch/1 -> Delay One Step2/1
  Delay One Step2/1 -> Relational Operator1/1, Switch1/1
  Switch1/1 -> Cntr/1, Switch/3, Increment Real World/1
  Relational Operator1/1 -> Switch1/2
  2/1 -> Switch1/3
  Max Value + 1/1 -> Relational Operator1/2
  Increment Real World/1 -> Switch/1
  Inc?/1 -> Switch/2

== matlab function OscillatorAndLockin_DynamicFreqMod/MATLAB Function1 ==
  data: SeparationDistance input; Force output; Potential output
%% Calculates the interaction Force and Potential as a function of seperation distance
function [Force,Potential] = TipSampleInteraction(SeparationDistance)
[Force,Potential] = sampledistanceLJ(SeparationDistance);
